simulink model "wutwut"  (R2014b)
settings: Solver=ode45  StartTime=0.0  StopTime=100.0  RelTol=1e-3
undefined symbols (not defined in the file): mian, s, s2, s3, s4, s5, wolny
settings Model: Creator=Jacek  LastModifiedBy=Jacek

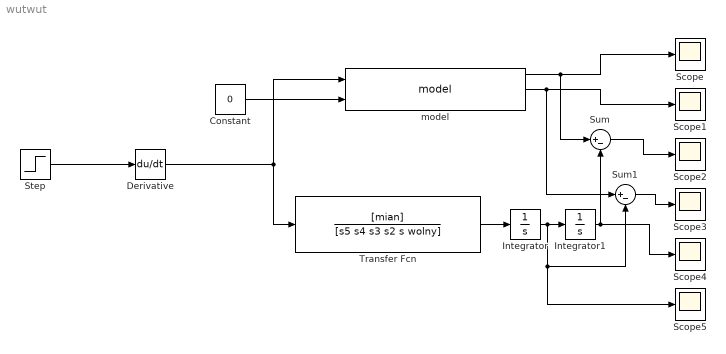
== system wutwut ==
  Constant : Constant  Value=0
  Derivative : Derivative
  Integrator : Integrator
  Integrator1 : Integrator
  Scope{,1..5} (6 alike) : Scope
      Scope2 settings: SaveName=ScopeData2
      Scope3 settings: SaveName=ScopeData3
      Scope4 settings: SaveName=ScopeData4
      Scope5 settings: SaveName=ScopeData5
  Step : Step  SampleTime=0
  Sum : Sum  Inputs=|+-
  Sum1 : Sum  Inputs=|+-
  Transfer Fcn : TransferFcn  Numerator=[mian]  Denominator=[s5 s4 s3 s2 s wolny]
  model : S-Function  FunctionName=model  EnableBusSupport=off
      mask Display: port_label('input',1,'Ein.'); port_label('input',2,'Fin.'); port_label('output',1,'Pout.'); port_label('output',2,'Vout.'); port_label('output',3,'DEBUG')
  wires:
  Derivative/1 -> Transfer Fcn/1, model/1
  Constant/1 -> model/2
  model/1 -> Sum/1, Scope/1
  model/2 -> Sum1/1, Scope1/1
  Integrator/1 -> Scope5/1, Sum1/2, Integrator1/1
  Transfer Fcn/1 -> Integrator/1
  Integrator1/1 -> Scope4/1, Sum/2
  Sum1/1 -> Scope3/1
  Sum/1 -> Scope2/1
  Step/1 -> Derivative/1
